simulink model "Chambers2010"  (Simulink 7.5)
settings: Solver=ode45  StartTime=0.0  StopTime=300  MaxStep=0.1  RelTol=1e-10
settings Model: Creator=Jordan  LastModifiedBy=jordan
settings OptimizationCC: InitFltsAndDblsToZero=on
settings DebuggingCC: SaveWithParameterizedLinksMsg=none  SignalResolutionControl=TryResolveAllWithWarning  MultiTaskDSMMsg=warning  MultiTaskCondExecSysMsg=none  StrictBusMsg=Warning
settings RTWCC: IncludeERTFirstTime=on
settings GRTTargetCC: TargetFcnLib=ansi_tfl_tmw.mat

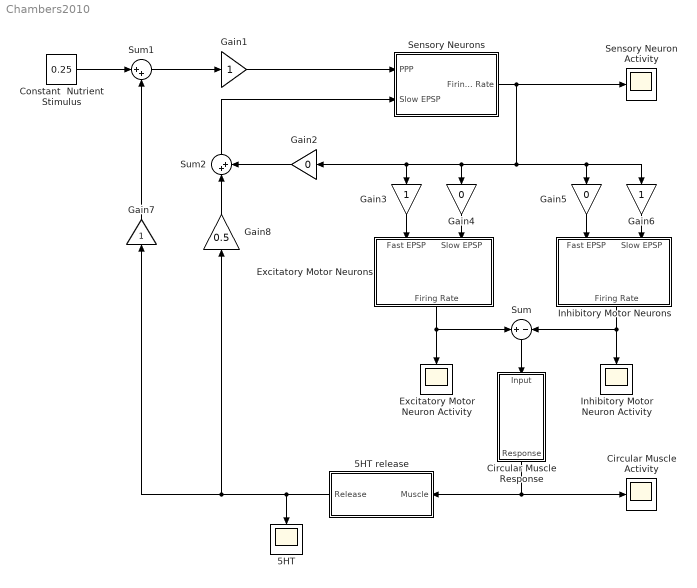
== system Chambers2010 ==
  5HT : Scope
      settings: SaveName=Serotonin_release  DataFormat=Array
  5HT release : Subsystem
  Circular Muscle Response : Subsystem
  Circular Muscle Activity : Scope
      settings: YMin=0  YMax=0.65  SaveName=Circular_Muscle  DataFormat=Array
  Constant  Nutrient Stimulus : Constant  Value=0.25  OutDataType=sfix(16)  OutScaling=2^0
  Excitatory Motor Neurons : Subsystem
  Excitatory Motor Neuron Activity : Scope
      settings: SaveName=Excitatory_Motor_Neurons  DataFormat=Array
  Gain{1,3,6..7} (4 alike) : Gain  ParameterDataType=sfix(16)  ParameterScaling=2^0  OutDataType=sfix(16)  OutScaling=2^0
  Gain2 : Gain  Gain=0  ParameterDataType=sfix(16)  ParameterScaling=2^0  OutDataType=sfix(16)  OutScaling=2^0
  Gain4 : Gain  Gain=0  ParameterDataType=sfix(16)  ParameterScaling=2^0  OutDataType=sfix(16)  OutScaling=2^0
  Gain5 : Gain  Gain=0  ParameterDataType=sfix(16)  ParameterScaling=2^0  OutDataType=sfix(16)  OutScaling=2^0
  Gain8 : Gain  Gain=0.5  ParameterDataType=sfix(16)  ParameterScaling=2^0  OutDataType=sfix(16)  OutScaling=2^0
  Inhibitory Motor Neurons : Subsystem
  Inhibitory Motor Neuron Activity : Scope
      settings: SaveName=Inhbitory_Motor_Neurons  DataFormat=Array
  Sensory Neuron Activity : Scope
      settings: YMin=0  YMax=1  SaveName=Sensory_Neurons  DataFormat=Array
  Sensory Neurons : Subsystem
  Sum : Sum  Inputs=+|-  OutDataType=sfix(16)  OutScaling=2^0
  Sum1 : Sum  Inputs=|++  OutDataType=sfix(16)  OutScaling=2^0
  Sum2 : Sum  Inputs=|++  OutDataType=sfix(16)  OutScaling=2^0
  wires:
  Sensory Neurons/1(Firing Rate) -> Sensory Neuron Activity/1, Gain2/1, Gain3/1, Gain4/1, Gain6/1, Gain5/1
  Gain1/1 -> Sensory Neurons/1(PPP)
  Constant  Nutrient Stimulus/1 -> Sum1/1
  Sum1/1 -> Gain1/1
  5HT release/1(Release) -> 5HT/1, Gain7/1, Gain8/1
  Sum2/1 -> Sensory Neurons/2(Slow EPSP)
  Gain2/1 -> Sum2/2
  Gain7/1 -> Sum1/2
  Excitatory Motor Neurons/1(Firing Rate) -> Sum/1, Excitatory Motor Neuron Activity/1
  Inhibitory Motor Neurons/1(Firing Rate) -> Sum/2, Inhibitory Motor Neuron Activity/1
  Circular Muscle Response/1(Response) -> 5HT release/1(Muscle), Circular Muscle Activity/1
  Sum/1 -> Circular Muscle Response/1(Input)
  Gain3/1 -> Excitatory Motor Neurons/1(Fast EPSP)
  Gain4/1 -> Excitatory Motor Neurons/2(Slow EPSP)
  Gain5/1 -> Inhibitory Motor Neurons/1(Fast EPSP)
  Gain6/1 -> Inhibitory Motor Neurons/2(Slow EPSP)
  Gain8/1 -> Sum2/1

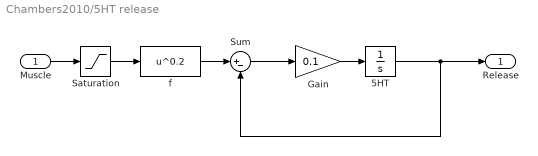
== system Chambers2010/5HT release ==
  Muscle : Inport  OutDataType=sfix(16)  OutScaling=2^0
  5HT : Integrator
  Gain : Gain  Gain=0.1  ParameterDataType=sfix(16)  ParameterScaling=2^0  OutDataType=sfix(16)  OutScaling=2^0
  Saturation : Saturate  UpperLimit=1  LowerLimit=0  LinearizeAsGain=off  ZeroCross=off
  Sum : Sum  Inputs=|+-  OutDataType=sfix(16)  OutScaling=2^0
  f : Fcn  Expr=u^0.2
  Release : Outport  OutDataType=sfix(16)  OutScaling=2^0
  wires:
  Muscle/1 -> Saturation/1
  f/1 -> Sum/1
  5HT/1 -> Release/1, Sum/2
  Sum/1 -> Gain/1
  Gain/1 -> 5HT/1
  Saturation/1 -> f/1

== system Chambers2010/Circular Muscle Response ==
  Input : Inport  OutDataType=sfix(16)  OutScaling=2^0
  Muscle : Integrator
  Sum1 : Sum  Inputs=|+-  OutDataType=sfix(16)  OutScaling=2^0
  Response : Outport  OutDataType=sfix(16)  OutScaling=2^0
  wires:
  Muscle/1 -> Response/1, Sum1/2
  Input/1 -> Sum1/1
  Sum1/1 -> Muscle/1

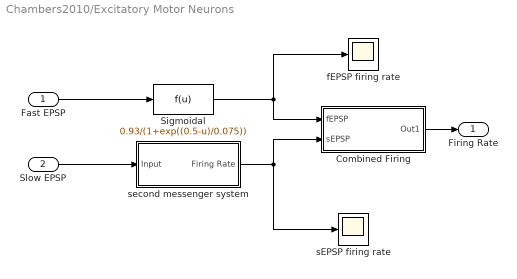
== system Chambers2010/Excitatory Motor Neurons ==
  Fast EPSP : Inport  OutDataType=sfix(16)  OutScaling=2^0
  Slow EPSP : Inport  Port=2  OutDataType=sfix(16)  OutScaling=2^0
  Combined Firing : Subsystem
  Sigmoidal : Fcn  Expr=0.93/(1+exp((0.5-u)/0.075))
  fEPSP firing rate : Scope
      settings: SaveName=ScopeData2
  sEPSP firing rate : Scope
  second messenger system : Subsystem
  Firing Rate : Outport  OutDataType=sfix(16)  OutScaling=2^0
  wires:
  Fast EPSP/1 -> Sigmoidal/1
  Slow EPSP/1 -> second messenger system/1(Input)
  Combined Firing/1(Out1) -> Firing Rate/1
  Sigmoidal/1 -> Combined Firing/1(fEPSP), fEPSP firing rate/1
  second messenger system/1(Firing Rate) -> Combined Firing/2(sEPSP), sEPSP firing rate/1

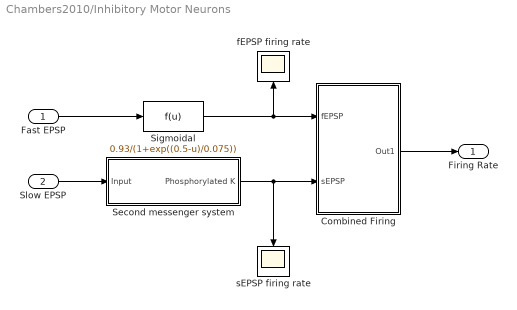
== system Chambers2010/Inhibitory Motor Neurons ==
  Fast EPSP : Inport  OutDataType=sfix(16)  OutScaling=2^0
  Slow EPSP : Inport  Port=2  OutDataType=sfix(16)  OutScaling=2^0
  Combined Firing : Subsystem
  Second messenger system : Subsystem
  Sigmoidal : Fcn  Expr=0.93/(1+exp((0.5-u)/0.075))
  fEPSP firing rate : Scope
      settings: SaveName=ScopeData2
  sEPSP firing rate : Scope
  Firing Rate : Outport  OutDataType=sfix(16)  OutScaling=2^0
  wires:
  Fast EPSP/1 -> Sigmoidal/1
  Slow EPSP/1 -> Second messenger system/1(Input)
  Combined Firing/1(Out1) -> Firing Rate/1
  Sigmoidal/1 -> Combined Firing/1(fEPSP), fEPSP firing rate/1
  Second messenger system/1(Phosphorylated K) -> Combined Firing/2(sEPSP), sEPSP firing rate/1

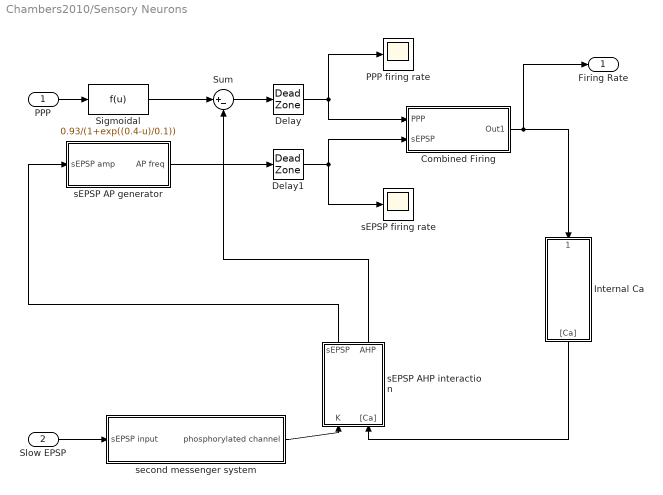
== system Chambers2010/Sensory Neurons ==
  PPP : Inport  OutDataType=sfix(16)  OutScaling=2^0
  Slow EPSP : Inport  Port=2  OutDataType=sfix(16)  OutScaling=2^0
  Combined Firing : Subsystem
  Delay : DeadZone  LowerValue=-1000  UpperValue=0.017  SaturateOnIntegerOverflow=on
  Delay1 : DeadZone  LowerValue=-1000  UpperValue=0  SaturateOnIntegerOverflow=on
  Internal Ca : Subsystem
  PPP firing rate : Scope
      settings: SaveName=fEPSPFR  DataFormat=Array
  Sigmoidal : Fcn  Expr=0.93/(1+exp((0.4-u)/0.1))
  Sum : Sum  Inputs=|+-  OutDataType=sfix(16)  OutScaling=2^0
  sEPSP AHP interaction : Subsystem
  sEPSP AP generator : Subsystem
  sEPSP firing rate : Scope
  second messenger system : Subsystem
  Firing Rate : Outport  OutDataType=sfix(16)  OutScaling=2^0
  wires:
  PPP/1 -> Sigmoidal/1
  Slow EPSP/1 -> second messenger system/1(sEPSP input)
  Combined Firing/1(Out1) -> Internal Ca/1(Firing rate), Firing Rate/1
  Sigmoidal/1 -> Sum/1
  Sum/1 -> Delay/1
  Delay/1 -> PPP firing rate/1, Combined Firing/1(PPP)
  second messenger system/1(phosphorylated channel) -> sEPSP AHP interaction/1(K)
  Internal Ca/1("[Ca]") -> sEPSP AHP interaction/2("[Ca]")
  sEPSP AHP interaction/1(sEPSP) -> sEPSP AP generator/1(sEPSP amp)
  Delay1/1 -> Combined Firing/2(sEPSP), sEPSP firing rate/1
  sEPSP AP generator/1(AP freq) -> Delay1/1
  sEPSP AHP interaction/2(AHP) -> Sum/2

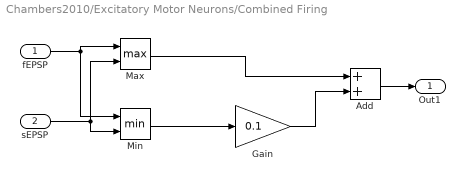
== system Chambers2010/Excitatory Motor Neurons/Combined Firing ==
  fEPSP : Inport  OutDataType=sfix(16)  OutScaling=2^0
  sEPSP : Inport  Port=2  OutDataType=sfix(16)  OutScaling=2^0
  Add : Sum  OutDataType=sfix(16)  OutScaling=2^-10
  Gain : Gain  Gain=0.1  ParameterDataType=sfix(16)  ParameterScaling=2^0  OutDataType=sfix(16)  OutScaling=2^0
  Max : MinMax  Function=max  Inputs=2  OutDataType=sfix(16)  OutScaling=2^0
  Min : MinMax  Inputs=2  OutDataType=sfix(16)  OutScaling=2^0
  Out1 : Outport  OutDataType=sfix(16)  OutScaling=2^0
  wires:
  fEPSP/1 -> Min/1, Max/1
  sEPSP/1 -> Max/2, Min/2
  Max/1 -> Add/1
  Min/1 -> Gain/1
  Gain/1 -> Add/2
  Add/1 -> Out1/1

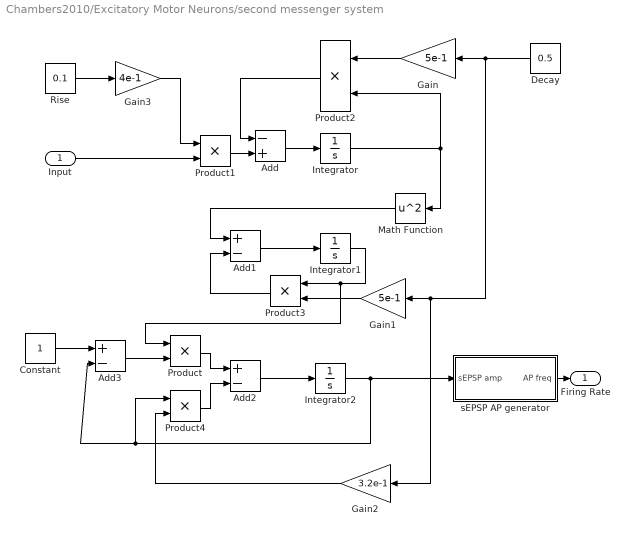
== system Chambers2010/Excitatory Motor Neurons/second messenger system ==
  Input : Inport  OutDataType=sfix(16)  OutScaling=2^0
  Add : Sum  Inputs=-+  OutDataType=sfix(16)  OutScaling=2^-10
  Add1 : Sum  Inputs=+-  OutDataType=sfix(16)  OutScaling=2^-10
  Add2 : Sum  Inputs=+-  OutDataType=sfix(16)  OutScaling=2^-10
  Add3 : Sum  Inputs=+-  OutDataType=sfix(16)  OutScaling=2^-10
  Constant : Constant  OutDataType=sfix(16)  OutScaling=2^0
  Decay : Constant  Value=0.5  OutDataType=sfix(16)  OutScaling=2^0
  Gain : Gain  Gain=5e-1  ParameterDataType=sfix(16)  ParameterScaling=2^0  OutDataType=sfix(16)  OutScaling=2^0
  Gain1 : Gain  Gain=5e-1  ParameterDataType=sfix(16)  ParameterScaling=2^0  OutDataType=sfix(16)  OutScaling=2^0
  Gain2 : Gain  Gain=3.2e-1  ParameterDataType=sfix(16)  ParameterScaling=2^0  OutDataType=sfix(16)  OutScaling=2^0
  Gain3 : Gain  Gain=4e-1  ParameterDataType=sfix(16)  ParameterScaling=2^0  OutDataType=sfix(16)  OutScaling=2^0
  Integrator : Integrator
  Integrator1 : Integrator
  Integrator2 : Integrator
  Math Function : Math  Operator=square  OutDataType=sfix(16)  OutScaling=2^0  SaturateOnIntegerOverflow=on
  Product : Product  OutDataType=sfix(16)  OutScaling=2^0  RndMeth=Zero
  Product1 : Product  Inputs=**  OutDataType=sfix(16)  OutScaling=2^-10
  Product2 : Product  Inputs=**  OutDataType=sfix(16)  OutScaling=2^-10
  Product3 : Product  OutDataType=sfix(16)  OutScaling=2^0  RndMeth=Zero
  Product4 : Product  OutDataType=sfix(16)  OutScaling=2^0  RndMeth=Zero
  Rise : Constant  Value=0.1  OutDataType=sfix(16)  OutScaling=2^0
  sEPSP AP generator : Subsystem
  Firing Rate : Outport  OutDataType=sfix(16)  OutScaling=2^0
  wires:
  Integrator/1 -> Product2/2, Math Function/1
  Add/1 -> Integrator/1
  Rise/1 -> Gain3/1
  Decay/1 -> Gain2/1, Gain1/1, Gain/1
  Product2/1 -> Add/1
  Product1/1 -> Add/2
  Add1/1 -> Integrator1/1
  Integrator1/1 -> Product3/1, Product/1
  Integrator2/1 -> Add3/2, Product4/1, sEPSP AP generator/1(sEPSP amp)
  Constant/1 -> Add3/1
  Product/1 -> Add2/1
  Add2/1 -> Integrator2/1
  Product3/1 -> Add1/2
  Product4/1 -> Add2/2
  Add3/1 -> Product/2
  Gain/1 -> Product2/1
  Gain1/1 -> Product3/2
  Gain2/1 -> Product4/2
  Gain3/1 -> Product1/1
  Math Function/1 -> Add1/1
  Input/1 -> Product1/2
  sEPSP AP generator/1(AP freq) -> Firing Rate/1

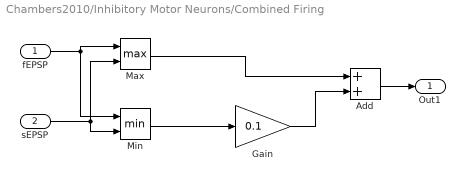
== system Chambers2010/Inhibitory Motor Neurons/Combined Firing ==
  fEPSP : Inport  OutDataType=sfix(16)  OutScaling=2^0
  sEPSP : Inport  Port=2  OutDataType=sfix(16)  OutScaling=2^0
  Add : Sum  OutDataType=sfix(16)  OutScaling=2^-10
  Gain : Gain  Gain=0.1  ParameterDataType=sfix(16)  ParameterScaling=2^0  OutDataType=sfix(16)  OutScaling=2^0
  Max : MinMax  Function=max  Inputs=2  OutDataType=sfix(16)  OutScaling=2^0
  Min : MinMax  Inputs=2  OutDataType=sfix(16)  OutScaling=2^0
  Out1 : Outport  OutDataType=sfix(16)  OutScaling=2^0
  wires:
  fEPSP/1 -> Min/1, Max/1
  sEPSP/1 -> Max/2, Min/2
  Max/1 -> Add/1
  Min/1 -> Gain/1
  Gain/1 -> Add/2
  Add/1 -> Out1/1

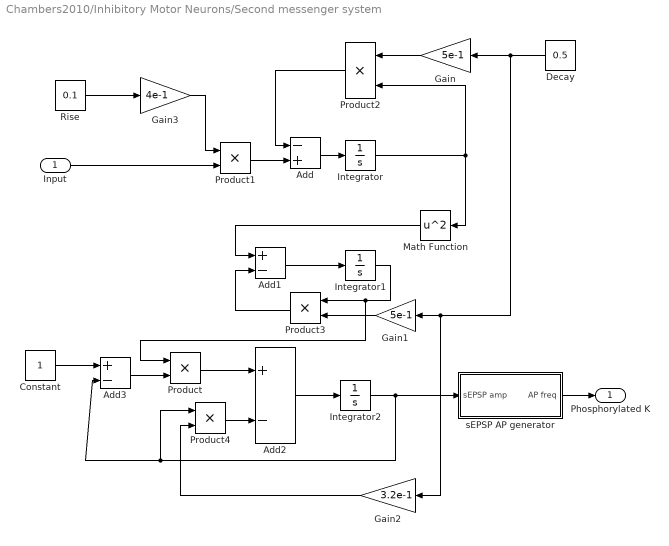
== system Chambers2010/Inhibitory Motor Neurons/Second messenger system ==
  Input : Inport  OutDataType=sfix(16)  OutScaling=2^0
  Add : Sum  Inputs=-+  OutDataType=sfix(16)  OutScaling=2^-10
  Add1 : Sum  Inputs=+-  OutDataType=sfix(16)  OutScaling=2^-10
  Add2 : Sum  Inputs=+-  OutDataType=sfix(16)  OutScaling=2^-10
  Add3 : Sum  Inputs=+-  OutDataType=sfix(16)  OutScaling=2^-10
  Constant : Constant  OutDataType=sfix(16)  OutScaling=2^0
  Decay : Constant  Value=0.5  OutDataType=sfix(16)  OutScaling=2^0
  Gain : Gain  Gain=5e-1  ParameterDataType=sfix(16)  ParameterScaling=2^0  OutDataType=sfix(16)  OutScaling=2^0
  Gain1 : Gain  Gain=5e-1  ParameterDataType=sfix(16)  ParameterScaling=2^0  OutDataType=sfix(16)  OutScaling=2^0
  Gain2 : Gain  Gain=3.2e-1  ParameterDataType=sfix(16)  ParameterScaling=2^0  OutDataType=sfix(16)  OutScaling=2^0
  Gain3 : Gain  Gain=4e-1  ParameterDataType=sfix(16)  ParameterScaling=2^0  OutDataType=sfix(16)  OutScaling=2^0
  Integrator : Integrator
  Integrator1 : Integrator
  Integrator2 : Integrator
  Math Function : Math  Operator=square  OutDataType=sfix(16)  OutScaling=2^0  SaturateOnIntegerOverflow=on
  Product : Product  OutDataType=sfix(16)  OutScaling=2^0  RndMeth=Zero
  Product1 : Product  Inputs=**  OutDataType=sfix(16)  OutScaling=2^-10
  Product2 : Product  Inputs=**  OutDataType=sfix(16)  OutScaling=2^-10
  Product3 : Product  OutDataType=sfix(16)  OutScaling=2^0  RndMeth=Zero
  Product4 : Product  OutDataType=sfix(16)  OutScaling=2^0  RndMeth=Zero
  Rise : Constant  Value=0.1  OutDataType=sfix(16)  OutScaling=2^0
  sEPSP AP generator : Subsystem
  Phosphorylated K : Outport  OutDataType=sfix(16)  OutScaling=2^0
  wires:
  Integrator/1 -> Product2/2, Math Function/1
  Add/1 -> Integrator/1
  Rise/1 -> Gain3/1
  Decay/1 -> Gain2/1, Gain1/1, Gain/1
  Product2/1 -> Add/1
  Product1/1 -> Add/2
  Add1/1 -> Integrator1/1
  Integrator1/1 -> Product3/1, Product/1
  Integrator2/1 -> Add3/2, Product4/1, sEPSP AP generator/1(sEPSP amp)
  Product/1 -> Add2/1
  Add2/1 -> Integrator2/1
  Product3/1 -> Add1/2
  Product4/1 -> Add2/2
  Add3/1 -> Product/2
  Gain/1 -> Product2/1
  Gain1/1 -> Product3/2
  Gain2/1 -> Product4/2
  Gain3/1 -> Product1/1
  Math Function/1 -> Add1/1
  Input/1 -> Product1/2
  sEPSP AP generator/1(AP freq) -> Phosphorylated K/1
  Constant/1 -> Add3/1

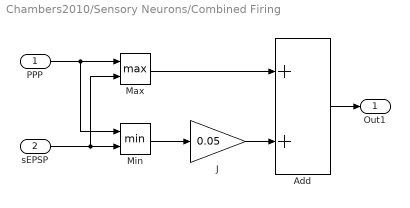
== system Chambers2010/Sensory Neurons/Combined Firing ==
  PPP : Inport  OutDataType=sfix(16)  OutScaling=2^0
  sEPSP : Inport  Port=2  OutDataType=sfix(16)  OutScaling=2^0
  Add : Sum  OutDataType=sfix(16)  OutScaling=2^-10
  J : Gain  Gain=0.05  ParameterDataType=sfix(16)  ParameterScaling=2^0  OutDataType=sfix(16)  OutScaling=2^0
  Max : MinMax  Function=max  Inputs=2  OutDataType=sfix(16)  OutScaling=2^0
  Min : MinMax  Inputs=2  OutDataType=sfix(16)  OutScaling=2^0
  Out1 : Outport  OutDataType=sfix(16)  OutScaling=2^0
  wires:
  PPP/1 -> Min/1, Max/1
  sEPSP/1 -> Max/2, Min/2
  Max/1 -> Add/1
  Min/1 -> J/1
  J/1 -> Add/2
  Add/1 -> Out1/1

== system Chambers2010/Sensory Neurons/Internal Ca ==
  Firing rate : Inport  OutDataType=sfix(16)  OutScaling=2^0
  AHP : Scope
      settings: SaveName=AHP  DataFormat=Array
  Ca entry (K) : Gain  ParameterDataType=sfix(16)  ParameterScaling=2^0  OutDataType=sfix(16)  OutScaling=2^0
  Calcium : Integrator
  Decay rate : Gain  ParameterDataType=sfix(16)  ParameterScaling=2^0  OutDataType=sfix(16)  OutScaling=2^0
  Sum1 : Sum  Inputs=|+-  OutDataType=sfix(16)  OutScaling=2^0
  "[Ca]" : Outport  OutDataType=sfix(16)  OutScaling=2^0
  wires:
  Firing rate/1 -> Ca entry (K)/1
  Calcium/1 -> AHP/1, Decay rate/1, "[Ca]"/1
  Sum1/1 -> Calcium/1
  Ca entry (K)/1 -> Sum1/1
  Decay rate/1 -> Sum1/2

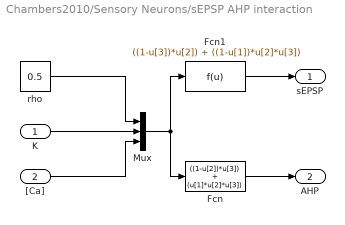
== system Chambers2010/Sensory Neurons/sEPSP AHP interaction ==
  K : Inport  OutDataType=sfix(16)  OutScaling=2^0
  "[Ca]" : Inport  Port=2  OutDataType=sfix(16)  OutScaling=2^0
  Fcn : Fcn  Expr=((1-u[2])*u[3]) + (u[1]*u[2]*u[3])
  Fcn1 : Fcn  Expr=((1-u[3])*u[2]) + ((1-u[1])*u[2]*u[3])
  Mux : Mux  Inputs=3
  rho : Constant  Value=0.5  OutDataType=sfix(16)  OutScaling=2^0
  sEPSP : Outport  OutDataType=sfix(16)  OutScaling=2^0
  AHP : Outport  Port=2  OutDataType=sfix(16)  OutScaling=2^0
  wires:
  Mux/1 -> Fcn/1, Fcn1/1
  rho/1 -> Mux/1
  K/1 -> Mux/2
  "[Ca]"/1 -> Mux/3
  Fcn/1 -> AHP/1
  Fcn1/1 -> sEPSP/1

== system Chambers2010/Sensory Neurons/sEPSP AP generator ==
  sEPSP amp : Inport  OutDataType=sfix(16)  OutScaling=2^0
  sEPSP APs : Fcn  Expr=(0.6/(1+exp((0.1-u)/0.003))) *(u^0.25)
  AP freq : Outport  OutDataType=sfix(16)  OutScaling=2^0
  wires:
  sEPSP amp/1 -> sEPSP APs/1
  sEPSP APs/1 -> AP freq/1

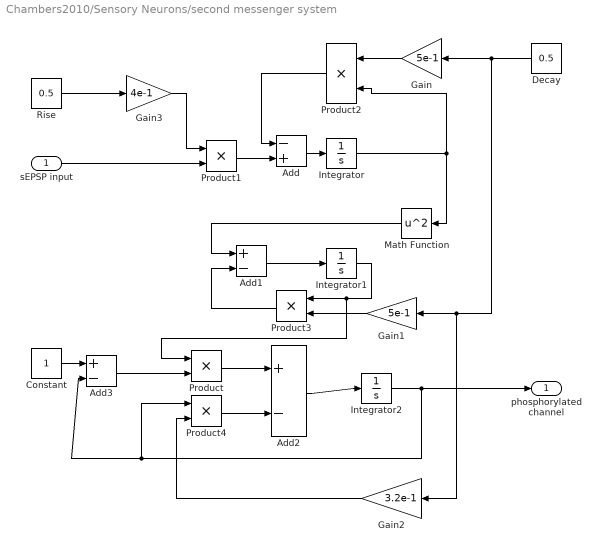
== system Chambers2010/Sensory Neurons/second messenger system ==
  sEPSP input : Inport  OutDataType=sfix(16)  OutScaling=2^0
  Add : Sum  Inputs=-+  OutDataType=sfix(16)  OutScaling=2^-10
  Add1 : Sum  Inputs=+-  OutDataType=sfix(16)  OutScaling=2^-10
  Add2 : Sum  Inputs=+-  OutDataType=sfix(16)  OutScaling=2^-10
  Add3 : Sum  Inputs=+-  OutDataType=sfix(16)  OutScaling=2^-10
  Constant : Constant  OutDataType=sfix(16)  OutScaling=2^0
  Decay : Constant  Value=0.5  OutDataType=sfix(16)  OutScaling=2^0
  Gain : Gain  Gain=5e-1  ParameterDataType=sfix(16)  ParameterScaling=2^0  OutDataType=sfix(16)  OutScaling=2^0
  Gain1 : Gain  Gain=5e-1  ParameterDataType=sfix(16)  ParameterScaling=2^0  OutDataType=sfix(16)  OutScaling=2^0
  Gain2 : Gain  Gain=3.2e-1  ParameterDataType=sfix(16)  ParameterScaling=2^0  OutDataType=sfix(16)  OutScaling=2^0
  Gain3 : Gain  Gain=4e-1  ParameterDataType=sfix(16)  ParameterScaling=2^0  OutDataType=sfix(16)  OutScaling=2^0
  Integrator : Integrator
  Integrator1 : Integrator
  Integrator2 : Integrator
  Math Function : Math  Operator=square  OutDataType=sfix(16)  OutScaling=2^0  SaturateOnIntegerOverflow=on
  Product : Product  OutDataType=sfix(16)  OutScaling=2^0  RndMeth=Zero
  Product1 : Product  Inputs=**  OutDataType=sfix(16)  OutScaling=2^-10
  Product2 : Product  Inputs=**  OutDataType=sfix(16)  OutScaling=2^-10
  Product3 : Product  OutDataType=sfix(16)  OutScaling=2^0  RndMeth=Zero
  Product4 : Product  OutDataType=sfix(16)  OutScaling=2^0  RndMeth=Zero
  Rise : Constant  Value=0.5  OutDataType=sfix(16)  OutScaling=2^0
  phosphorylated channel : Outport  OutDataType=sfix(16)  OutScaling=2^0
  wires:
  Integrator/1 -> Product2/2, Math Function/1
  Add/1 -> Integrator/1
  Rise/1 -> Gain3/1
  Decay/1 -> Gain2/1, Gain1/1, Gain/1
  Product2/1 -> Add/1
  Product1/1 -> Add/2
  Add1/1 -> Integrator1/1
  Integrator1/1 -> Product3/1, Product/1
  Integrator2/1 -> Add3/2, Product4/1, phosphorylated channel/1
  Constant/1 -> Add3/1
  Product/1 -> Add2/1
  Add2/1 -> Integrator2/1
  Product3/1 -> Add1/2
  Product4/1 -> Add2/2
  Add3/1 -> Product/2
  Gain/1 -> Product2/1
  Gain1/1 -> Product3/2
  Gain2/1 -> Product4/2
  Gain3/1 -> Product1/1
  Math Function/1 -> Add1/1
  sEPSP input/1 -> Product1/2

== system Chambers2010/Excitatory Motor Neurons/second messenger system/sEPSP AP generator ==
  sEPSP amp : Inport  OutDataType=sfix(16)  OutScaling=2^0
  Saturation : Saturate  UpperLimit=10000  LowerLimit=0
  sEPSP APs : Fcn  Expr=(1/(1+exp((0.1-u)/0.02))) *(u^0.25)
  AP freq : Outport  OutDataType=sfix(16)  OutScaling=2^0
  wires:
  sEPSP amp/1 -> Saturation/1
  sEPSP APs/1 -> AP freq/1
  Saturation/1 -> sEPSP APs/1

== system Chambers2010/Inhibitory Motor Neurons/Second messenger system/sEPSP AP generator ==
  sEPSP amp : Inport  OutDataType=sfix(16)  OutScaling=2^0
  Saturation : Saturate  UpperLimit=10000  LowerLimit=0
  sEPSP APs : Fcn  Expr=(1/(1+exp((0.1-u)/0.02))) *(u^0.25)
  AP freq : Outport  OutDataType=sfix(16)  OutScaling=2^0
  wires:
  sEPSP amp/1 -> Saturation/1
  sEPSP APs/1 -> AP freq/1
  Saturation/1 -> sEPSP APs/1
